simulink model "CompareControllers"  (R2020b)
settings: Solver=ode45  StartTime=0.0  StopTime=2  RelTol=1e-3
undefined symbols (not defined in the file or in its folder): daq, degs2rpm, ees, es, io, pid, robust, rpm2rads, sens, ss
libraries: simulink x1
settings Model: Creator=Utente  LastModifiedBy=Utente

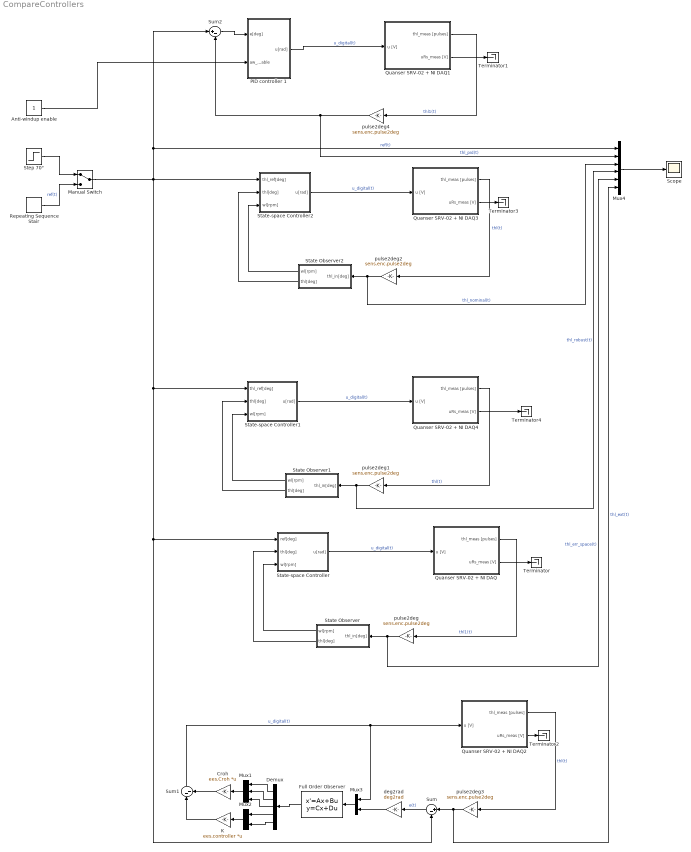
== system CompareControllers ==
  Anti-windup enable : Constant
  Croh : Gain  Gain=ees.Croh  Multiplication=Matrix(K*u)
  Demux : Demux  Outputs=5
  Full Order Observer : StateSpace  A=ees.Ae4 - ees.estimator4.Le*ees.Ce  B=[ees.Be, ees.estimator4.Le]  C=eye(5)  D=[0,0;0,0;0,0;0,0;0,0]  InitialCondition=0
  K : Gain  Gain=ees.controller  Multiplication=Matrix(K*u)
  Manual Switch : ManualSwitch
  Mux1 : Mux  Inputs=3
  Mux2 : Mux  Inputs=2
  Mux3 : Mux  Inputs=2
  Mux4 : Mux  Inputs=6
  PID controller 1 : Subsystem
  Quanser SRV-02 + NI DAQ : Subsystem  mask(Quanser SRV-02 (with inertial load) + NI DAQ){Ts=0.001, fricType=Karnopp}
      mask prompts: Ts "NI DAQ Sample Time:"; fricType "Friction model"
      mask help: Quanser SRV-02 (with inertial load) + NI DAQ model.
      mask init:
      | %%  Sensors data
      | 
      | %   shunt resistor
      | sens.curr.Rs = 0.5;                         %   resistance [Ohm]   
      | sens.curr.uRs_std = 0.01;                   %   voltage noise standard dev [V]                           
      | sens.curr.uRs_var = sens.curr.uRs_std^2;	%   voltage noise variance [V^2]
      | 
      | %   Hewlett-Packard HEDS-5540#A06 optical encoder
      | sens.enc.ppr = 500*4;                       %   pulses per rotation
      | sens.enc.pulse2deg = 360/sens.enc.ppr;      %   [pulses] -> [deg]
      | sens.enc.pulse2rad = 2*pi/sens.enc.ppr;     %   [pulses] -> [rad]
      | sens.enc.deg2pulse = sens.enc.ppr/360;      %   [deg] -> [pulses]
      | sens.enc.rad2pulse = sens.enc.ppr/2/pi;     %   [rad] -> [pulses]
      | 
      | 
      | %%  Data acquisition board (daq) data
      | 
      | %   NI PCI-6221 DAC data
      | daq.dac.bits = 16;                                  %   resolution (bits)
      | daq.dac.fs   = 10;                                  %   full scale 
      | daq.dac.q    = 2*daq.dac.fs/(2^daq.dac.bits-1);     %	quantization
      | 
      | %   NI PCI-6221 ADC data
      | daq.adc.bits = 16;                                  %   resolution (bits)
      | daq.adc.fs   = 10;                                  %   full scale (as set in SLDRT Analog Input block)
      | daq.adc.q    = 2*daq.adc.fs/(2^daq.adc.bits-1);     %   quantization
      mask Help:
      | Riccardo Antonello (antonello@dei.unipd.it)
      | 
      | April 24, 2020
      | 
      | Dept. of Information Engineering, University of Padova
      mask TypeOptions fricType: Coulomb + viscous | Karnopp
  Quanser SRV-02 + NI DAQ1 : Subsystem  mask(Quanser SRV-02 (with inertial load) + NI DAQ){Ts=0.001, fricType=Karnopp}
      mask prompts: Ts "NI DAQ Sample Time:"; fricType "Friction model"
      mask help: Quanser SRV-02 (with inertial load) + NI DAQ model.
      mask init: same as CompareControllers/Quanser SRV-02 + NI DAQ
      mask Help:
      | Riccardo Antonello (antonello@dei.unipd.it)
      | 
      | April 24, 2020
      | 
      | Dept. of Information Engineering, University of Padova
      mask TypeOptions fricType: Coulomb + viscous | Karnopp
  Quanser SRV-02 + NI DAQ2 : Subsystem  mask(Quanser SRV-02 (with inertial load) + NI DAQ){Ts=0.001, fricType=Karnopp}
      mask prompts: Ts "NI DAQ Sample Time:"; fricType "Friction model"
      mask help: Quanser SRV-02 (with inertial load) + NI DAQ model.
      mask init: same as CompareControllers/Quanser SRV-02 + NI DAQ
      mask Help:
      | Riccardo Antonello (antonello@dei.unipd.it)
      | 
      | April 24, 2020
      | 
      | Dept. of Information Engineering, University of Padova
      mask TypeOptions fricType: Coulomb + viscous | Karnopp
  Quanser SRV-02 + NI DAQ3 : Subsystem  mask(Quanser SRV-02 (with inertial load) + NI DAQ){Ts=0.001, fricType=Karnopp}
      mask prompts: Ts "NI DAQ Sample Time:"; fricType "Friction model"
      mask help: Quanser SRV-02 (with inertial load) + NI DAQ model.
      mask init: same as CompareControllers/Quanser SRV-02 + NI DAQ
      mask Help:
      | Riccardo Antonello (antonello@dei.unipd.it)
      | 
      | April 24, 2020
      | 
      | Dept. of Information Engineering, University of Padova
      mask TypeOptions fricType: Coulomb + viscous | Karnopp
  Quanser SRV-02 + NI DAQ4 : Subsystem  mask(Quanser SRV-02 (with inertial load) + NI DAQ){Ts=0.001, fricType=Karnopp}
      mask prompts: Ts "NI DAQ Sample Time:"; fricType "Friction model"
      mask help: Quanser SRV-02 (with inertial load) + NI DAQ model.
      mask init: same as CompareControllers/Quanser SRV-02 + NI DAQ
      mask Help:
      | Riccardo Antonello (antonello@dei.unipd.it)
      | 
      | April 24, 2020
      | 
      | Dept. of Information Engineering, University of Padova
      mask TypeOptions fricType: Coulomb + viscous | Karnopp
  Repeating Sequence Stair : simulink/Sources/Repeating Sequence Stair  OutValues=[30 0 70 0 90].'  tsamp=1  OutMin=[]  OutMax=[]  OutDataTypeStr=double  OutputDataTypeScalingMode=double  OutDataType=fixdt(0,8)  ConRadixGroup=Best Precision: Vector-wise  OutScaling=2^-12
  Scope : Scope
  State Observer : Subsystem
  State Observer1 : Subsystem
  State Observer2 : Subsystem
  State-space Controller : Subsystem
  State-space Controller1 : Subsystem
  State-space Controller2 : Subsystem
  Step 70° : Step  Time=0  After=70  SampleTime=0
  Sum : Sum  Inputs=|+-
  Sum1 : Sum  Inputs=|--
  Sum2 : Sum  Inputs=|+-
  Terminator{,1..4} (5 alike) : Terminator
  deg2rad : Gain  Gain=deg2rad
  pulse2deg{,1..4} (5 alike) : Gain  Gain=sens.enc.pulse2deg
  wires:
  State Observer/2(thl[deg]) -> State-space Controller/2(thl[deg])
  State Observer/1(wl[rpm]) -> State-space Controller/3(wl[rpm])
  pulse2deg/1 -> Mux4/5, State Observer/1(thl_in[deg])  "thl_err_space(t)"
  State-space Controller/1(u[rad]) -> Quanser SRV-02 + NI DAQ/1(u [V])  "u_digital(t)"
  Quanser SRV-02 + NI DAQ/1(thl_meas [pulses]) -> pulse2deg/1  "thl1(t)"
  Quanser SRV-02 + NI DAQ/2(uRs_meas [V]) -> Terminator/1
  State-space Controller1/1(u[rad]) -> Quanser SRV-02 + NI DAQ4/1(u [V])  "u_digital(t)"
  Quanser SRV-02 + NI DAQ4/1(thl_meas [pulses]) -> pulse2deg1/1  "thl(t)"
  State Observer1/2(thl[deg]) -> State-space Controller1/2(thl[deg])
  pulse2deg1/1 -> Mux4/4, State Observer1/1(thl_in[deg])  "thl_robust(t)"
  State Observer1/1(wl[rpm]) -> State-space Controller1/3(wl[rpm])
  pulse2deg2/1 -> Mux4/3, State Observer2/1(thl_in[deg])  "thl_nominal(t)"
  State Observer2/2(thl[deg]) -> State-space Controller2/2(thl[deg])
  State Observer2/1(wl[rpm]) -> State-space Controller2/3(wl[rpm])
  Quanser SRV-02 + NI DAQ3/1(thl_meas [pulses]) -> pulse2deg2/1  "thl(t)"
  State-space Controller2/1(u[rad]) -> Quanser SRV-02 + NI DAQ3/1(u [V])  "u_digital(t)"
  Full Order Observer/1 -> Demux/1
  K/1 -> Sum1/1
  Croh/1 -> Sum1/2
  Mux3/1 -> Full Order Observer/1
  deg2rad/1 -> Mux3/2
  Demux/5 -> Mux2/2
  Sum/1 -> deg2rad/1  "e(t)"
  pulse2deg3/1 -> Mux4/6, Sum/1  "thl_ext(t)"
  Demux/3 -> Mux1/3
  Mux2/1 -> K/1
  Sum1/1 -> Quanser SRV-02 + NI DAQ2/1(u [V]), Mux3/1  "u_digital(t)"
  Quanser SRV-02 + NI DAQ2/1(thl_meas [pulses]) -> pulse2deg3/1  "thl(t)"
  Demux/2 -> Mux1/2
  Demux/1 -> Mux1/1
  Mux1/1 -> Croh/1
  Demux/4 -> Mux2/1
  Quanser SRV-02 + NI DAQ1/1(thl_meas [pulses]) -> pulse2deg4/1  "thl1(t)"
  Quanser SRV-02 + NI DAQ1/2(uRs_meas [V]) -> Terminator1/1
  Sum2/1 -> PID controller 1/1(e[deg])
  pulse2deg4/1 -> Mux4/2, Sum2/2  "thl_pid(t)"
  Quanser SRV-02 + NI DAQ2/2(uRs_meas [V]) -> Terminator2/1
  Quanser SRV-02 + NI DAQ3/2(uRs_meas [V]) -> Terminator3/1
  Quanser SRV-02 + NI DAQ4/2(uRs_meas [V]) -> Terminator4/1
  Mux4/1 -> Scope/1
  Manual Switch/1 -> State-space Controller2/1(thl_ref[deg]), State-space Controller1/1(thl_ref[deg]), Sum/2, State-space Controller/1(ref[deg]), Sum2/1, Mux4/1  "ref(t)"
  Repeating Sequence Stair/1 -> Manual Switch/2  "ref(t)"
  Step 70°/1 -> Manual Switch/1
  PID controller 1/1(u[rad]) -> Quanser SRV-02 + NI DAQ1/1(u [V])  "u_digital(t)"
  Anti-windup enable/1 -> PID controller 1/2(aw_enable)

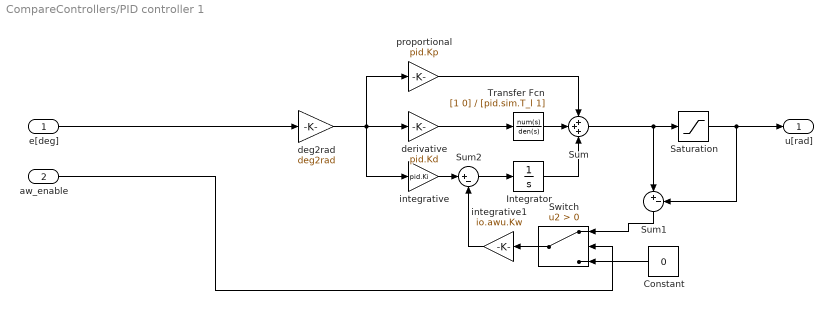
== system CompareControllers/PID controller 1 ==
  e[deg] : Inport  Unit=deg
  aw_enable : Inport  Port=2  Unit=deg
  Constant : Constant  Value=0
  Integrator : Integrator
  Saturation : Saturate  UpperLimit=daq.dac.vdd  LowerLimit=daq.dac.vss
  Sum : Sum  Inputs=+++
  Sum1 : Sum  Inputs=|+-
  Sum2 : Sum  Inputs=|+-
  Switch : Switch  Criteria=u2 > Threshold
  Transfer Fcn : TransferFcn  Numerator=[1 0]  Denominator=[pid.sim.T_l 1]
  deg2rad : Gain  Gain=deg2rad
  derivative : Gain  Gain=pid.Kd
  integrative : Gain  Gain=pid.Ki
  integrative1 : Gain  Gain=io.awu.Kw
  proportional : Gain  Gain=pid.Kp
  u[rad] : Outport
  wires:
  deg2rad/1 -> integrative/1, derivative/1, proportional/1
  proportional/1 -> Sum/1
  Saturation/1 -> Sum1/2, u[rad]/1
  integrative/1 -> Sum2/1
  Sum2/1 -> Integrator/1
  integrative1/1 -> Sum2/2
  Integrator/1 -> Sum/3
  Transfer Fcn/1 -> Sum/2
  derivative/1 -> Transfer Fcn/1
  aw_enable/1 -> Switch/2
  Constant/1 -> Switch/3
  Switch/1 -> integrative1/1
  Sum1/1 -> Switch/1
  Sum/1 -> Saturation/1, Sum1/1
  e[deg]/1 -> deg2rad/1

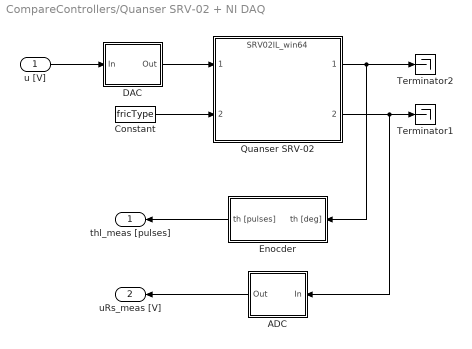
== system CompareControllers/Quanser SRV-02 + NI DAQ ==
  u [V] : Inport
  ADC : Subsystem
  Constant : Constant  Value=fricType
  DAC : Subsystem
  Enocder : Subsystem
  Quanser SRV-02 : ModelReference  ModelNameDialog=SRV02IL_win64.slxp  ModelReferenceVersion=1.44  CopyOfModelProtected=on
  Terminator1 : Terminator
  Terminator2 : Terminator
  thl_meas [pulses] : Outport
  uRs_meas [V] : Outport  Port=2
  wires:
  Enocder/1(th [pulses]) -> thl_meas [pulses]/1
  ADC/1(Out) -> uRs_meas [V]/1
  DAC/1(Out) -> Quanser SRV-02/1
  Quanser SRV-02/2 -> ADC/1(In), Terminator1/1
  u [V]/1 -> DAC/1(In)
  Quanser SRV-02/1 -> Enocder/1(th [deg]), Terminator2/1
  Constant/1 -> Quanser SRV-02/2

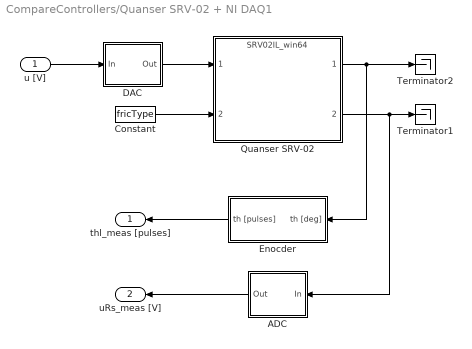
== system CompareControllers/Quanser SRV-02 + NI DAQ1 ==
  u [V] : Inport
  ADC : Subsystem
  Constant : Constant  Value=fricType
  DAC : Subsystem
  Enocder : Subsystem
  Quanser SRV-02 : ModelReference  ModelNameDialog=SRV02IL_win64.slxp  ModelReferenceVersion=1.44  CopyOfModelProtected=on
  Terminator1 : Terminator
  Terminator2 : Terminator
  thl_meas [pulses] : Outport
  uRs_meas [V] : Outport  Port=2
  wires:
  Enocder/1(th [pulses]) -> thl_meas [pulses]/1
  ADC/1(Out) -> uRs_meas [V]/1
  DAC/1(Out) -> Quanser SRV-02/1
  Quanser SRV-02/2 -> ADC/1(In), Terminator1/1
  u [V]/1 -> DAC/1(In)
  Quanser SRV-02/1 -> Enocder/1(th [deg]), Terminator2/1
  Constant/1 -> Quanser SRV-02/2

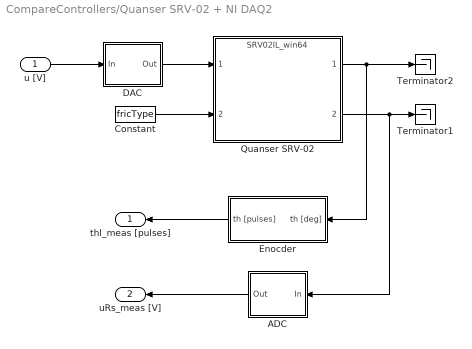
== system CompareControllers/Quanser SRV-02 + NI DAQ2 ==
  u [V] : Inport
  ADC : Subsystem
  Constant : Constant  Value=fricType
  DAC : Subsystem
  Enocder : Subsystem
  Quanser SRV-02 : ModelReference  ModelNameDialog=SRV02IL_win64.slxp  ModelReferenceVersion=1.44  CopyOfModelProtected=on
  Terminator1 : Terminator
  Terminator2 : Terminator
  thl_meas [pulses] : Outport
  uRs_meas [V] : Outport  Port=2
  wires:
  Enocder/1(th [pulses]) -> thl_meas [pulses]/1
  ADC/1(Out) -> uRs_meas [V]/1
  DAC/1(Out) -> Quanser SRV-02/1
  Quanser SRV-02/2 -> ADC/1(In), Terminator1/1
  u [V]/1 -> DAC/1(In)
  Quanser SRV-02/1 -> Enocder/1(th [deg]), Terminator2/1
  Constant/1 -> Quanser SRV-02/2

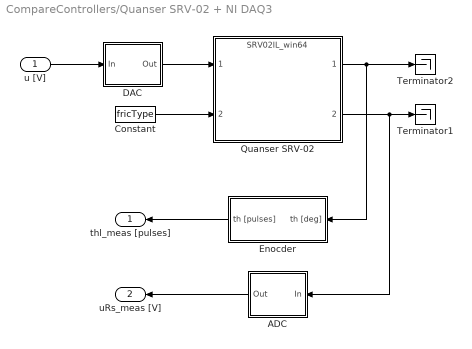
== system CompareControllers/Quanser SRV-02 + NI DAQ3 ==
  u [V] : Inport
  ADC : Subsystem
  Constant : Constant  Value=fricType
  DAC : Subsystem
  Enocder : Subsystem
  Quanser SRV-02 : ModelReference  ModelNameDialog=SRV02IL_win64.slxp  ModelReferenceVersion=1.44  CopyOfModelProtected=on
  Terminator1 : Terminator
  Terminator2 : Terminator
  thl_meas [pulses] : Outport
  uRs_meas [V] : Outport  Port=2
  wires:
  Enocder/1(th [pulses]) -> thl_meas [pulses]/1
  ADC/1(Out) -> uRs_meas [V]/1
  DAC/1(Out) -> Quanser SRV-02/1
  Quanser SRV-02/2 -> ADC/1(In), Terminator1/1
  u [V]/1 -> DAC/1(In)
  Quanser SRV-02/1 -> Enocder/1(th [deg]), Terminator2/1
  Constant/1 -> Quanser SRV-02/2

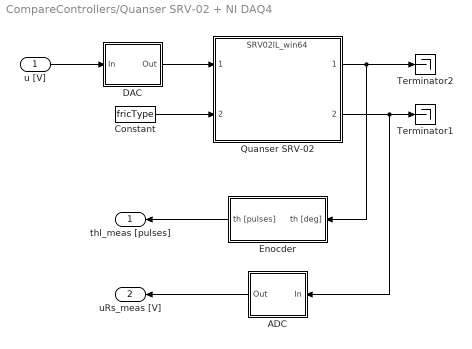
== system CompareControllers/Quanser SRV-02 + NI DAQ4 ==
  u [V] : Inport
  ADC : Subsystem
  Constant : Constant  Value=fricType
  DAC : Subsystem
  Enocder : Subsystem
  Quanser SRV-02 : ModelReference  ModelNameDialog=SRV02IL_win64.slxp  ModelReferenceVersion=1.44  CopyOfModelProtected=on
  Terminator1 : Terminator
  Terminator2 : Terminator
  thl_meas [pulses] : Outport
  uRs_meas [V] : Outport  Port=2
  wires:
  Enocder/1(th [pulses]) -> thl_meas [pulses]/1
  ADC/1(Out) -> uRs_meas [V]/1
  DAC/1(Out) -> Quanser SRV-02/1
  Quanser SRV-02/2 -> ADC/1(In), Terminator1/1
  u [V]/1 -> DAC/1(In)
  Quanser SRV-02/1 -> Enocder/1(th [deg]), Terminator2/1
  Constant/1 -> Quanser SRV-02/2

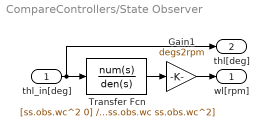
== system CompareControllers/State Observer ==
  thl_in[deg] : Inport
  Gain1 : Gain  Gain=degs2rpm
  Transfer Fcn : TransferFcn  Numerator=[ss.obs.wc^2 0]  Denominator=[1 2*ss.obs.delta*ss.obs.wc ss.obs.wc^2]
  wl[rpm] : Outport
  thl[deg] : Outport  Port=2
  wires:
  Transfer Fcn/1 -> Gain1/1
  thl_in[deg]/1 -> thl[deg]/1, Transfer Fcn/1
  Gain1/1 -> wl[rpm]/1

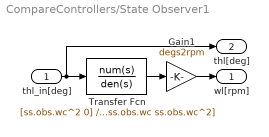
== system CompareControllers/State Observer1 ==
  thl_in[deg] : Inport
  Gain1 : Gain  Gain=degs2rpm
  Transfer Fcn : TransferFcn  Numerator=[ss.obs.wc^2 0]  Denominator=[1 2*ss.obs.delta*ss.obs.wc ss.obs.wc^2]
  wl[rpm] : Outport
  thl[deg] : Outport  Port=2
  wires:
  Transfer Fcn/1 -> Gain1/1
  thl_in[deg]/1 -> thl[deg]/1, Transfer Fcn/1
  Gain1/1 -> wl[rpm]/1

== system CompareControllers/State Observer2 ==
  thl_in[deg] : Inport
  Gain1 : Gain  Gain=degs2rpm
  Transfer Fcn : TransferFcn  Numerator=[ss.obs.wc^2 0]  Denominator=[1 2*ss.obs.delta*ss.obs.wc ss.obs.wc^2]
  wl[rpm] : Outport
  thl[deg] : Outport  Port=2
  wires:
  Transfer Fcn/1 -> Gain1/1
  thl_in[deg]/1 -> thl[deg]/1, Transfer Fcn/1
  Gain1/1 -> wl[rpm]/1

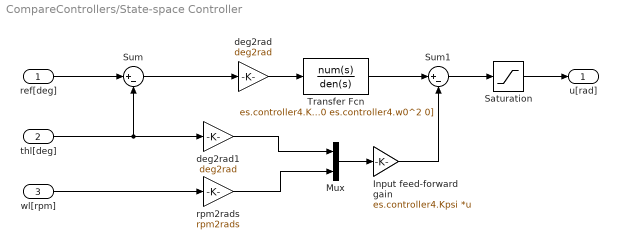
== system CompareControllers/State-space Controller ==
  ref[deg] : Inport
  thl[deg] : Inport  Port=2
  wl[rpm] : Inport  Port=3
  Input feed-forward gain : Gain  Gain=es.controller4.Kpsi  Multiplication=Matrix(K*u)
  Mux : Mux  Inputs=2
  Saturation : Saturate  UpperLimit=daq.dac.vdd  LowerLimit=daq.dac.vss
  Sum : Sum  Inputs=|+-
  Sum1 : Sum  Inputs=|+-
  Transfer Fcn : TransferFcn  Numerator=es.controller4.Kz  Denominator=[1 0 es.controller4.w0^2 0]
  deg2rad : Gain  Gain=deg2rad
  deg2rad1 : Gain  Gain=deg2rad
  rpm2rads : Gain  Gain=rpm2rads
  u[rad] : Outport
  wires:
  rpm2rads/1 -> Mux/2
  deg2rad1/1 -> Mux/1
  Saturation/1 -> u[rad]/1
  wl[rpm]/1 -> rpm2rads/1
  thl[deg]/1 -> Sum/2, deg2rad1/1
  deg2rad/1 -> Transfer Fcn/1
  Transfer Fcn/1 -> Sum1/1
  Input feed-forward gain/1 -> Sum1/2
  Mux/1 -> Input feed-forward gain/1
  Sum1/1 -> Saturation/1
  Sum/1 -> deg2rad/1
  ref[deg]/1 -> Sum/1

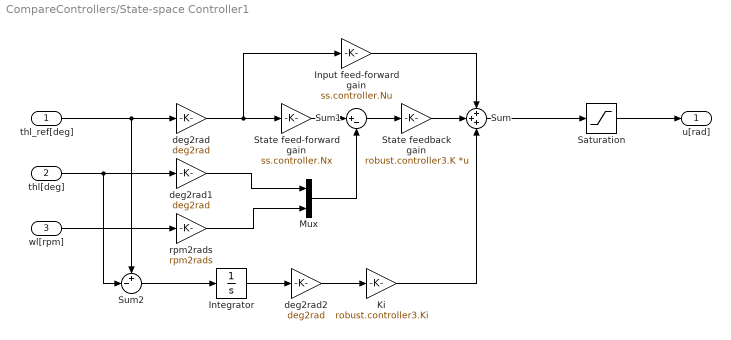
== system CompareControllers/State-space Controller1 ==
  thl_ref[deg] : Inport
  thl[deg] : Inport  Port=2
  wl[rpm] : Inport  Port=3
  Input feed-forward gain : Gain  Gain=ss.controller.Nu
  Integrator : Integrator
  Ki : Gain  Gain=robust.controller3.Ki
  Mux : Mux  Inputs=2
  Saturation : Saturate  UpperLimit=daq.dac.vdd  LowerLimit=daq.dac.vss
  State feed-forward gain : Gain  Gain=ss.controller.Nx
  State feedback gain : Gain  Gain=robust.controller3.K  Multiplication=Matrix(K*u)
  Sum : Sum  Inputs=+++
  Sum1 : Sum  Inputs=|+-
  Sum2 : Sum  Inputs=+-|
  deg2rad : Gain  Gain=deg2rad
  deg2rad1 : Gain  Gain=deg2rad
  deg2rad2 : Gain  Gain=deg2rad
  rpm2rads : Gain  Gain=rpm2rads
  u[rad] : Outport
  wires:
  rpm2rads/1 -> Mux/2
  Sum1/1 -> State feedback gain/1
  Mux/1 -> Sum1/2
  thl_ref[deg]/1 -> Sum2/1, deg2rad/1
  deg2rad/1 -> Input feed-forward gain/1, State feed-forward gain/1
  State feed-forward gain/1 -> Sum1/1
  deg2rad1/1 -> Mux/1
  Input feed-forward gain/1 -> Sum/1
  Saturation/1 -> u[rad]/1
  wl[rpm]/1 -> rpm2rads/1
  thl[deg]/1 -> Sum2/2, deg2rad1/1
  State feedback gain/1 -> Sum/2
  Sum/1 -> Saturation/1
  Sum2/1 -> Integrator/1
  Integrator/1 -> deg2rad2/1
  deg2rad2/1 -> Ki/1
  Ki/1 -> Sum/3

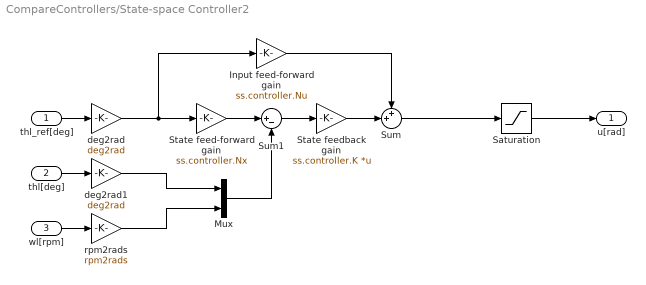
== system CompareControllers/State-space Controller2 ==
  thl_ref[deg] : Inport
  thl[deg] : Inport  Port=2
  wl[rpm] : Inport  Port=3
  Input feed-forward gain : Gain  Gain=ss.controller.Nu
  Mux : Mux  Inputs=2
  Saturation : Saturate  UpperLimit=daq.dac.vdd  LowerLimit=daq.dac.vss
  State feed-forward gain : Gain  Gain=ss.controller.Nx
  State feedback gain : Gain  Gain=ss.controller.K  Multiplication=Matrix(K*u)
  Sum : Sum  Inputs=++|
  Sum1 : Sum  Inputs=|+-
  deg2rad : Gain  Gain=deg2rad
  deg2rad1 : Gain  Gain=deg2rad
  rpm2rads : Gain  Gain=rpm2rads
  u[rad] : Outport
  wires:
  rpm2rads/1 -> Mux/2
  Sum1/1 -> State feedback gain/1
  Mux/1 -> Sum1/2
  thl_ref[deg]/1 -> deg2rad/1
  deg2rad/1 -> Input feed-forward gain/1, State feed-forward gain/1
  State feed-forward gain/1 -> Sum1/1
  deg2rad1/1 -> Mux/1
  Input feed-forward gain/1 -> Sum/1
  Saturation/1 -> u[rad]/1
  wl[rpm]/1 -> rpm2rads/1
  thl[deg]/1 -> deg2rad1/1
  State feedback gain/1 -> Sum/2
  Sum/1 -> Saturation/1

== system CompareControllers/Quanser SRV-02 + NI DAQ/ADC ==
  In : Inport
  Quantizer : Quantizer  QuantizationInterval=daq.adc.q
  Saturation : Saturate  UpperLimit=daq.adc.fs  LowerLimit=-daq.adc.fs
  Zero-Order Hold : ZeroOrderHold  SampleTime=Ts
  Out : Outport
  wires:
  Saturation/1 -> Out/1
  In/1 -> Zero-Order Hold/1
  Quantizer/1 -> Saturation/1
  Zero-Order Hold/1 -> Quantizer/1

== system CompareControllers/Quanser SRV-02 + NI DAQ/DAC ==
  In : Inport
  Quantizer : Quantizer  QuantizationInterval=daq.dac.q
  Saturation : Saturate  UpperLimit=daq.dac.fs  LowerLimit=-daq.dac.fs
  Zero-Order Hold : ZeroOrderHold  SampleTime=Ts
  Out : Outport
  wires:
  Quantizer/1 -> Saturation/1
  In/1 -> Zero-Order Hold/1
  Zero-Order Hold/1 -> Quantizer/1
  Saturation/1 -> Out/1

== system CompareControllers/Quanser SRV-02 + NI DAQ/Enocder ==
  th [deg] : Inport
  Quantizer : Quantizer  QuantizationInterval=sens.enc.pulse2deg
  Zero-Order Hold : ZeroOrderHold  SampleTime=Ts
  deg2pulse : Gain  Gain=sens.enc.deg2pulse
  th [pulses] : Outport
  wires:
  Quantizer/1 -> deg2pulse/1
  th [deg]/1 -> Zero-Order Hold/1
  Zero-Order Hold/1 -> Quantizer/1
  deg2pulse/1 -> th [pulses]/1

== system CompareControllers/Quanser SRV-02 + NI DAQ1/ADC ==
  In : Inport
  Quantizer : Quantizer  QuantizationInterval=daq.adc.q
  Saturation : Saturate  UpperLimit=daq.adc.fs  LowerLimit=-daq.adc.fs
  Zero-Order Hold : ZeroOrderHold  SampleTime=Ts
  Out : Outport
  wires:
  Saturation/1 -> Out/1
  In/1 -> Zero-Order Hold/1
  Quantizer/1 -> Saturation/1
  Zero-Order Hold/1 -> Quantizer/1

== system CompareControllers/Quanser SRV-02 + NI DAQ1/DAC ==
  In : Inport
  Quantizer : Quantizer  QuantizationInterval=daq.dac.q
  Saturation : Saturate  UpperLimit=daq.dac.fs  LowerLimit=-daq.dac.fs
  Zero-Order Hold : ZeroOrderHold  SampleTime=Ts
  Out : Outport
  wires:
  Quantizer/1 -> Saturation/1
  In/1 -> Zero-Order Hold/1
  Zero-Order Hold/1 -> Quantizer/1
  Saturation/1 -> Out/1

== system CompareControllers/Quanser SRV-02 + NI DAQ1/Enocder ==
  th [deg] : Inport
  Quantizer : Quantizer  QuantizationInterval=sens.enc.pulse2deg
  Zero-Order Hold : ZeroOrderHold  SampleTime=Ts
  deg2pulse : Gain  Gain=sens.enc.deg2pulse
  th [pulses] : Outport
  wires:
  Quantizer/1 -> deg2pulse/1
  th [deg]/1 -> Zero-Order Hold/1
  Zero-Order Hold/1 -> Quantizer/1
  deg2pulse/1 -> th [pulses]/1

== system CompareControllers/Quanser SRV-02 + NI DAQ2/ADC ==
  In : Inport
  Quantizer : Quantizer  QuantizationInterval=daq.adc.q
  Saturation : Saturate  UpperLimit=daq.adc.fs  LowerLimit=-daq.adc.fs
  Zero-Order Hold : ZeroOrderHold  SampleTime=Ts
  Out : Outport
  wires:
  Saturation/1 -> Out/1
  In/1 -> Zero-Order Hold/1
  Quantizer/1 -> Saturation/1
  Zero-Order Hold/1 -> Quantizer/1

== system CompareControllers/Quanser SRV-02 + NI DAQ2/DAC ==
  In : Inport
  Quantizer : Quantizer  QuantizationInterval=daq.dac.q
  Saturation : Saturate  UpperLimit=daq.dac.fs  LowerLimit=-daq.dac.fs
  Zero-Order Hold : ZeroOrderHold  SampleTime=Ts
  Out : Outport
  wires:
  Quantizer/1 -> Saturation/1
  In/1 -> Zero-Order Hold/1
  Zero-Order Hold/1 -> Quantizer/1
  Saturation/1 -> Out/1

== system CompareControllers/Quanser SRV-02 + NI DAQ2/Enocder ==
  th [deg] : Inport
  Quantizer : Quantizer  QuantizationInterval=sens.enc.pulse2deg
  Zero-Order Hold : ZeroOrderHold  SampleTime=Ts
  deg2pulse : Gain  Gain=sens.enc.deg2pulse
  th [pulses] : Outport
  wires:
  Quantizer/1 -> deg2pulse/1
  th [deg]/1 -> Zero-Order Hold/1
  Zero-Order Hold/1 -> Quantizer/1
  deg2pulse/1 -> th [pulses]/1

== system CompareControllers/Quanser SRV-02 + NI DAQ3/ADC ==
  In : Inport
  Quantizer : Quantizer  QuantizationInterval=daq.adc.q
  Saturation : Saturate  UpperLimit=daq.adc.fs  LowerLimit=-daq.adc.fs
  Zero-Order Hold : ZeroOrderHold  SampleTime=Ts
  Out : Outport
  wires:
  Saturation/1 -> Out/1
  In/1 -> Zero-Order Hold/1
  Quantizer/1 -> Saturation/1
  Zero-Order Hold/1 -> Quantizer/1

== system CompareControllers/Quanser SRV-02 + NI DAQ3/DAC ==
  In : Inport
  Quantizer : Quantizer  QuantizationInterval=daq.dac.q
  Saturation : Saturate  UpperLimit=daq.dac.fs  LowerLimit=-daq.dac.fs
  Zero-Order Hold : ZeroOrderHold  SampleTime=Ts
  Out : Outport
  wires:
  Quantizer/1 -> Saturation/1
  In/1 -> Zero-Order Hold/1
  Zero-Order Hold/1 -> Quantizer/1
  Saturation/1 -> Out/1

== system CompareControllers/Quanser SRV-02 + NI DAQ3/Enocder ==
  th [deg] : Inport
  Quantizer : Quantizer  QuantizationInterval=sens.enc.pulse2deg
  Zero-Order Hold : ZeroOrderHold  SampleTime=Ts
  deg2pulse : Gain  Gain=sens.enc.deg2pulse
  th [pulses] : Outport
  wires:
  Quantizer/1 -> deg2pulse/1
  th [deg]/1 -> Zero-Order Hold/1
  Zero-Order Hold/1 -> Quantizer/1
  deg2pulse/1 -> th [pulses]/1

== system CompareControllers/Quanser SRV-02 + NI DAQ4/ADC ==
  In : Inport
  Quantizer : Quantizer  QuantizationInterval=daq.adc.q
  Saturation : Saturate  UpperLimit=daq.adc.fs  LowerLimit=-daq.adc.fs
  Zero-Order Hold : ZeroOrderHold  SampleTime=Ts
  Out : Outport
  wires:
  Saturation/1 -> Out/1
  In/1 -> Zero-Order Hold/1
  Quantizer/1 -> Saturation/1
  Zero-Order Hold/1 -> Quantizer/1

== system CompareControllers/Quanser SRV-02 + NI DAQ4/DAC ==
  In : Inport
  Quantizer : Quantizer  QuantizationInterval=daq.dac.q
  Saturation : Saturate  UpperLimit=daq.dac.fs  LowerLimit=-daq.dac.fs
  Zero-Order Hold : ZeroOrderHold  SampleTime=Ts
  Out : Outport
  wires:
  Quantizer/1 -> Saturation/1
  In/1 -> Zero-Order Hold/1
  Zero-Order Hold/1 -> Quantizer/1
  Saturation/1 -> Out/1

== system CompareControllers/Quanser SRV-02 + NI DAQ4/Enocder ==
  th [deg] : Inport
  Quantizer : Quantizer  QuantizationInterval=sens.enc.pulse2deg
  Zero-Order Hold : ZeroOrderHold  SampleTime=Ts
  deg2pulse : Gain  Gain=sens.enc.deg2pulse
  th [pulses] : Outport
  wires:
  Quantizer/1 -> deg2pulse/1
  th [deg]/1 -> Zero-Order Hold/1
  Zero-Order Hold/1 -> Quantizer/1
  deg2pulse/1 -> th [pulses]/1
